simulink model "controller"  (R2022b)
settings: Solver=ode4  StartTime=0.0  StopTime=4  FixedStep=0.001  RelTol=1e-3
PreLoadFcn:
  | global m1 m2 l g m1_hat m2_hat;
  | m1 = 2;
  | m2 = 2;
  | m1_hat = 0.97*m1;
  | m2_hat = 0.97*m2;
  | l = 1;
  | g = 9.81;
  | 
  | kd = 200;
  | md = m1_hat;
  | dd = 2*0.7*sqrt(kd*md);
  | 
  | Kd = [kd,0;0,kd];
  | Md = [md,0;0,md];
  | Dd = [dd,0;0,dd];
  | 
  | p = 10^6;
  | d = 2*0.7*sqrt(p);
  | 
  | P = [p,0;0,p];
  | D = [d,0;0,d];
  | 
  | D_hold = D;
  | P_hold = P;
  | 
  | ke = 300;
  | Ke = [ke,0;0,0];
  | 
  | Fc = 1;
  | cv = 4;
  | 
  | delta = 0.01;
  | 
  | x0 = [0.95,0.95];
  | dx0 = [0;0];
  | 
  | n_pow = 0.001;
  | 
  | wall = 0.8;
  | 
  | delay = 2;
libraries: simulink x19, bbblueBasicLib x7
(part 1 of 2)
settings Model: SimulationMode=external  ExtModeTrigDuration=100  Creator=Nick  LastModifiedBy=ABL
settings SolverCC: PositivePriorityOrder=on  AutoInsertRateTranBlk=on  InsertRTBMode=Always
settings OptimizationCC: EnhancedBackFolding=on  PassReuseOutputArgsAs=Individual arguments  ZeroExternalMemoryAtStartup=off  ZeroInternalMemoryAtStartup=off  MaxStackSize=64  OptimizeBlockOrder=speed  DifferentSizesBufferReuse=on  OptimizationCustomize=off  EfficientTunableParamExpr=on
settings DebuggingCC: ParameterTunabilityLossMsg=error  UnconnectedInputMsg=warning  UnconnectedOutputMsg=warning  UnconnectedLineMsg=warning
settings HardwareCC: ProdBitPerPointer=32  ProdBitPerSizeT=32  ProdBitPerPtrDiffT=32  ProdLargestAtomicInteger=Long  ProdLargestAtomicFloat=Double  ProdWordSize=32  ProdHWDeviceType=ARM Compatible->ARM Cortex  UseEmbeddedCoderFeatures=off
settings ModelReferenceCC: EnableRefExpFcnMdlSchedulingChecks=on
settings SFSimCC: SimUserIncludeDirs=placeholders  MATLABDynamicMemAlloc=off
settings SFSimCC: SimCustomHeaderCode=|
  | #include "init_can.h"
  | #include "get_encoder.h"
  | #include "set_motor.h"
  | #include "print_input.h"
  | #include "stop_motor.h"
  | #include "datalog.h"
settings SFSimCC: SimUserSources=|
  | placeholders\init_can.c
  | placeholders\set_motor.c
  | placeholders\get_encoder.c
  | placeholders\print_input.c
  | placeholders\stop_motor.c
  | placeholders\datalog.c
settings RTWCC: Description=Embedded Coder  SystemTargetFile=ert.tlc  HardwareBoard=BeagleBone Blue  TLCOptions="-aInlineSetEventsForThisBaseRateFcn=TLC_FALSE -aSuppressMultiTaskScheduler=TLC_FALSE  -aRateBasedStepFcn=0"  TemplateMakefile=ert_default_tmf  RTWUseSimCustomCode=on  CustomInclude=placeholders  Toolchain=GNU GCC BeagleBone Blue  BuildConfiguration=Faster Runs  DLArmComputeVersion=19.05
settings RTWCC: CustomHeaderCode=|
  | #include "init_can.h"
  | #include "get_encoder.h"
  | #include "set_motor.h"
  | #include "print_input.h"
  | #include "stop_motor.h"
  | #include "datalog.h"
settings RTWCC: CustomSource=|
  | placeholders\init_can.c
  | placeholders\set_motor.c
  | placeholders\get_encoder.c
  | placeholders\print_input.c
  | placeholders\stop_motor.c
  | placeholders\datalog.c
settings CodeAppCC: ForceParamTrailComments=on  IgnoreCustomStorageClasses=off  OperatorAnnotations=on  SimulinkDataObjDesc=on  SFDataObjDesc=on  InsertBlockDesc=on
settings ERTTargetCC: SupportNonInlinedSFcns=on  SupportVariableSizeSignals=on

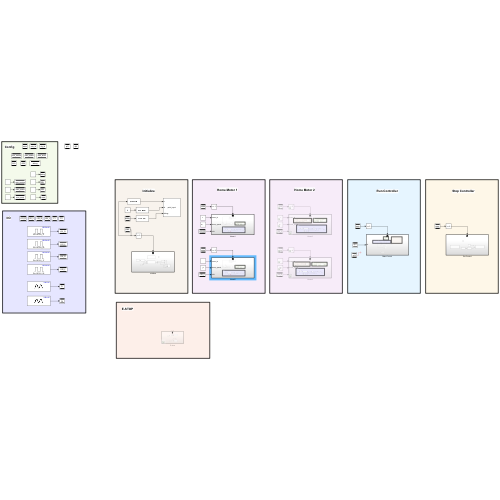
[thumbnail: Simulink's stored preview of the top-level diagram]
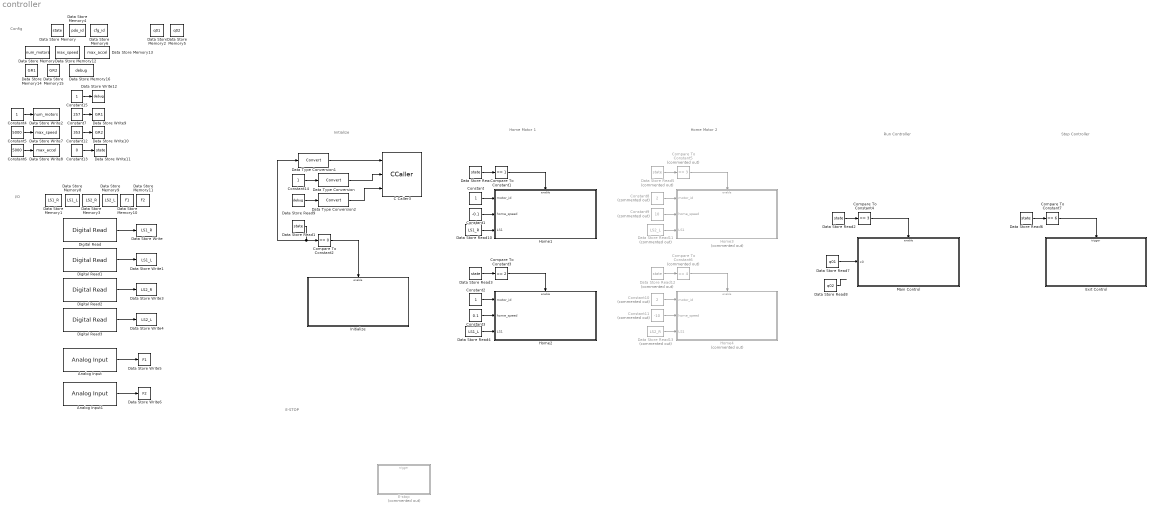
== system controller ==
  note: E-STOP
  note: Run Controller
  note: Home Motor 1
  note: Initialize
  note: Config
  note: I/O
  note: Stop Controller
  note: Home Motor 2
  Analog Input : bbblueBasicLib/Analog Input  Pin=AIN0  Mode=Raw  SampleTime=0.1  SimulateUsing=Code generation
  Analog Input1 : bbblueBasicLib/Analog Input  Pin=AIN0  Mode=Raw  SampleTime=0.1  SimulateUsing=Code generation
  C Caller3 : CCaller  FunctionName=print_input  PortSpecificationStruct="%)30     .    : 4   8    (     @         %    \"     ,    !     0         %  0 \"0    $    _    07)G3F%M90  4&]R=$YA;64 4V-O<&4     26YD97@     5'EP90      4VEZ90      27-';&]B86P   X    P    !@    @    $          4    (     0    $    !         !   0!A    #@   #     &    \"     0         !0    @    !     0    $         $  ! &$    .    .     8    (    !          %    \"     $    %     0         0    !0   $EN<'5T    #@   #@    &    \"     8         !0    @    !     0    $         \"0    @               X    X    !@    @    $          4    (     0    4    !         !     %    :6YT,S(    .    ,     8    (    !          %    \"     $    !     0         0  $ ,0    X    P    !@    @    ) @        4    (     0    $    !          (  0      #@   #     &    \"     0         !0    @    !     @    $         $  \" &ED   .    ,     8    (    !          %    \"     $    \"     0         0  ( :60   X    X    !@    @    $          4    (     0    4    !         !     %    26YP=70    .    .     8    (    !@         %    \"     $    !     0         )    \"            / _#@   #@    &    \"     0         !0    @    !    !0    $         $     4   !I;G0S,@    X    P    !@    @    $          4    (     0    $    !         !   0 Q    #@   #     &    \"     D\"        !0    @    !     0    $          @ !       .    .     8    (    !          %    \"     $    %     0         0    !0   &1E8G5G    #@   #@    &    \"     0         !0    @    !    !0    $         $     4   !D96)U9P    X    X    !@    @    $          4    (     0    4    !         !     %    26YP=70    .    .     8    (    !@         %    \"     $    !     0         )    \"             ! #@   #@    &    \"     0         !0    @    !    !0    $         $     4   !I;G0S,@    X    P    !@    @    $          4    (     0    $    !         !   0 Q    #@   #     &    \"     D\"        !0    @    !     0    $          @ !"  SampleTime=1
  Compare To Constant1 : simulink/Logic and Bit Operations/Compare To Constant  relop===  const=1  OutDataTypeStr=boolean
  Compare To Constant2 : simulink/Logic and Bit Operations/Compare To Constant  relop===  const=0  OutDataTypeStr=boolean
  Compare To Constant3 : simulink/Logic and Bit Operations/Compare To Constant  relop===  const=2  OutDataTypeStr=boolean
  Compare To Constant4 : simulink/Logic and Bit Operations/Compare To Constant  relop===  const=3  OutDataTypeStr=boolean
  Compare To Constant5 : simulink/Logic and Bit Operations/Compare To Constant  Commented=on  relop===  const=3  OutDataTypeStr=boolean
  Compare To Constant6 : simulink/Logic and Bit Operations/Compare To Constant  Commented=on  relop===  const=4  OutDataTypeStr=boolean
  Compare To Constant7 : simulink/Logic and Bit Operations/Compare To Constant  relop===  const=6  OutDataTypeStr=boolean
  Constant{,2,4,14..15} (5 alike) : Constant
  Constant1 : Constant  Value=-0.1
  Constant10 : Constant  Commented=on  Value=2
  Constant11 : Constant  Commented=on  Value=-10
  Constant12 : Constant  Value=353
  Constant13 : Constant  Value=0
  Constant3 : Constant  Value=0.1
  Constant5 : Constant  Value=5000
  Constant6 : Constant  Value=5000
  Constant7 : Constant  Value=257
  Constant8 : Constant  Commented=on  Value=2
  Constant9 : Constant  Commented=on  Value=10
  Data Store Memory : DataStoreMemory  DataStoreName=state  WriteAfterWriteMsg=warning  ShowAdditionalParam=off  OutDataTypeStr=double
  Data Store Memory1 : DataStoreMemory  DataStoreName=LS1_R  WriteAfterWriteMsg=warning  ShowAdditionalParam=off
  Data Store Memory10 : DataStoreMemory  DataStoreName=F1  WriteAfterWriteMsg=warning  ShowAdditionalParam=off
  Data Store Memory11 : DataStoreMemory  DataStoreName=F2  WriteAfterWriteMsg=warning  ShowAdditionalParam=off
  Data Store Memory12 : DataStoreMemory  DataStoreName=max_speed  WriteAfterWriteMsg=warning  ShowAdditionalParam=off
  Data Store Memory13 : DataStoreMemory  DataStoreName=max_accel  WriteAfterWriteMsg=warning  ShowAdditionalParam=off
  Data Store Memory14 : DataStoreMemory  DataStoreName=GR1  WriteAfterWriteMsg=warning  ShowAdditionalParam=off
  Data Store Memory15 : DataStoreMemory  DataStoreName=GR2  WriteAfterWriteMsg=warning  ShowAdditionalParam=off
  Data Store Memory16 : DataStoreMemory  DataStoreName=debug  WriteAfterWriteMsg=warning  ShowAdditionalParam=off
  Data Store Memory2 : DataStoreMemory  DataStoreName=q01  WriteAfterWriteMsg=warning  ShowAdditionalParam=off
  Data Store Memory3 : DataStoreMemory  DataStoreName=LS2_R  WriteAfterWriteMsg=warning  ShowAdditionalParam=off
  Data Store Memory4 : DataStoreMemory  DataStoreName=pdo_id  WriteAfterWriteMsg=warning  ShowAdditionalParam=off
  Data Store Memory5 : DataStoreMemory  DataStoreName=q02  WriteAfterWriteMsg=warning  ShowAdditionalParam=off
  Data Store Memory6 : DataStoreMemory  DataStoreName=cfg_id  WriteAfterWriteMsg=warning  ShowAdditionalParam=off
  Data Store Memory7 : DataStoreMemory  DataStoreName=num_motors  WriteAfterWriteMsg=warning  ShowAdditionalParam=off
  Data Store Memory8 : DataStoreMemory  DataStoreName=LS1_L  WriteAfterWriteMsg=warning  ShowAdditionalParam=off
  Data Store Memory9 : DataStoreMemory  DataStoreName=LS2_L  WriteAfterWriteMsg=warning  ShowAdditionalParam=off
  Data Store Read{,1..3,6} (5 alike) : DataStoreRead  DataStoreName=state  IndexOptions=Index vector (dialog)  Indices=1  OutputSizes=1
  Data Store Read10 : DataStoreRead  DataStoreName=LS1_R  IndexOptions=Index vector (dialog)  Indices=1  OutputSizes=1
  Data Store Read11 : DataStoreRead  Commented=on  DataStoreName=LS2_L  IndexOptions=Index vector (dialog)  Indices=1  OutputSizes=1
  Data Store Read12 : DataStoreRead  Commented=on  DataStoreName=state  IndexOptions=Index vector (dialog)  Indices=1  OutputSizes=1
  Data Store Read13 : DataStoreRead  Commented=on  DataStoreName=LS2_R  IndexOptions=Index vector (dialog)  Indices=1  OutputSizes=1
  Data Store Read4 : DataStoreRead  DataStoreName=LS1_L  IndexOptions=Index vector (dialog)  Indices=1  OutputSizes=1
  Data Store Read5 : DataStoreRead  Commented=on  DataStoreName=state  IndexOptions=Index vector (dialog)  Indices=1  OutputSizes=1
  Data Store Read7 : DataStoreRead  DataStoreName=q01  IndexOptions=Index vector (dialog)  Indices=1  OutputSizes=1
  Data Store Read8 : DataStoreRead  DataStoreName=q02  IndexOptions=Index vector (dialog)  Indices=1  OutputSizes=1
  Data Store Read9 : DataStoreRead  DataStoreName=debug  IndexOptions=Index vector (dialog)  Indices=1  OutputSizes=1
  Data Store Write : DataStoreWrite  DataStoreName=LS1_R  IndexOptions=Index vector (dialog)  Indices=1  OutputSizes=1
  Data Store Write1 : DataStoreWrite  DataStoreName=LS1_L  IndexOptions=Index vector (dialog)  Indices=1  OutputSizes=1
  Data Store Write10 : DataStoreWrite  DataStoreName=GR2  IndexOptions=Index vector (dialog)  Indices=1  OutputSizes=1
  Data Store Write11 : DataStoreWrite  DataStoreName=state  SampleTime=10000  IndexOptions=Index vector (dialog)  Indices=1  OutputSizes=1
  Data Store Write12 : DataStoreWrite  DataStoreName=debug  IndexOptions=Index vector (dialog)  Indices=1  OutputSizes=1
  Data Store Write2 : DataStoreWrite  DataStoreName=num_motors  IndexOptions=Index vector (dialog)  Indices=1  OutputSizes=1
  Data Store Write3 : DataStoreWrite  DataStoreName=LS2_R  IndexOptions=Index vector (dialog)  Indices=1  OutputSizes=1
  Data Store Write4 : DataStoreWrite  DataStoreName=LS2_L  IndexOptions=Index vector (dialog)  Indices=1  OutputSizes=1
  Data Store Write5 : DataStoreWrite  DataStoreName=F1  IndexOptions=Index vector (dialog)  Indices=1  OutputSizes=1
  Data Store Write6 : DataStoreWrite  DataStoreName=F2  IndexOptions=Index vector (dialog)  Indices=1  OutputSizes=1
  Data Store Write7 : DataStoreWrite  DataStoreName=max_speed  IndexOptions=Index vector (dialog)  Indices=1  OutputSizes=1
  Data Store Write8 : DataStoreWrite  DataStoreName=max_accel  IndexOptions=Index vector (dialog)  Indices=1  OutputSizes=1
  Data Store Write9 : DataStoreWrite  DataStoreName=GR1  IndexOptions=Index vector (dialog)  Indices=1  OutputSizes=1
  Data Type Conversion : DataTypeConversion  SaturateOnIntegerOverflow=off  RndMeth=Floor
  Data Type Conversion1 : DataTypeConversion  SaturateOnIntegerOverflow=off  RndMeth=Floor
  Data Type Conversion2 : DataTypeConversion  SaturateOnIntegerOverflow=off  RndMeth=Floor
  Digital Read : bbblueBasicLib/Digital Read  Pin=49  Direction=input  GPIOSelect=GPIO3_17  SampleTime=0.1
  Digital Read1 : bbblueBasicLib/Digital Read  Pin=49  Direction=input  GPIOSelect=GPIO3_20  SampleTime=0.1
  Digital Read2 : bbblueBasicLib/Digital Read  Pin=49  Direction=input  GPIOSelect=GPIO1_17  SampleTime=0.1
  Digital Read3 : bbblueBasicLib/Digital Read  Pin=49  Direction=input  GPIOSelect=GPIO1_25  SampleTime=0.1
  E-stop : Subsystem  Commented=on  TreatAsAtomicUnit=on
  Exit Control : Subsystem
  Home1 : Subsystem
  Home2 : Subsystem
  Home3 : Subsystem  Commented=on
  Home4 : Subsystem  Commented=on
  Initialize : Subsystem
  Main Control : Subsystem
  wires:
  Data Store Read/1 -> Compare To Constant1/1
  Compare To Constant1/1 -> Home1/Enable
  Compare To Constant2/1 -> Initialize/Enable
  Constant/1 -> Home1/1(motor_id)
  Constant1/1 -> Home1/2(home_speed)
  Data Store Read6/1 -> Compare To Constant7/1
  Compare To Constant7/1 -> Exit Control/Trigger
  Constant4/1 -> Data Store Write2/1
  Digital Read2/1 -> Data Store Write3/1
  Digital Read3/1 -> Data Store Write4/1
  Analog Input/1 -> Data Store Write5/1
  Analog Input1/1 -> Data Store Write6/1
  Constant5/1 -> Data Store Write7/1
  Constant6/1 -> Data Store Write8/1
  Data Store Read2/1 -> Compare To Constant4/1
  Compare To Constant4/1 -> Main Control/Enable
  Digital Read/1 -> Data Store Write/1
  Constant7/1 -> Data Store Write9/1
  Constant12/1 -> Data Store Write10/1
  Data Type Conversion/1 -> C Caller3/2
  Constant13/1 -> Data Store Write11/1
  Data Type Conversion1/1 -> C Caller3/1
  Digital Read1/1 -> Data Store Write1/1
  Data Store Read7/1 -> Main Control/1(x0)
  Data Store Read8/1 -> ?
  Constant15/1 -> Data Store Write12/1
  Constant14/1 -> Data Type Conversion/1
  Data Store Read9/1 -> Data Type Conversion2/1
  Data Type Conversion2/1 -> C Caller3/3
  Data Store Read10/1 -> Home1/3(LS1)
  Constant9/1 -> Home3/2(home_speed)
  Compare To Constant6/1 -> Home4/Enable
  Data Store Read13/1 -> Home4/3(LS1)
  Constant11/1 -> Home4/2(home_speed)
  Data Store Read11/1 -> Home3/3(LS1)
  Constant8/1 -> Home3/1(motor_id)
  Data Store Read12/1 -> Compare To Constant6/1
  Constant10/1 -> Home4/1(motor_id)
  Compare To Constant5/1 -> Home3/Enable
  Data Store Read5/1 -> Compare To Constant5/1
  Data Store Read1/1 -> Compare To Constant2/1, Data Type Conversion1/1
  Data Store Read3/1 -> Compare To Constant3/1
  Constant3/1 -> Home2/2(home_speed)
  Constant2/1 -> Home2/1(motor_id)
  Data Store Read4/1 -> Home2/3(LS1)
  Compare To Constant3/1 -> Home2/Enable

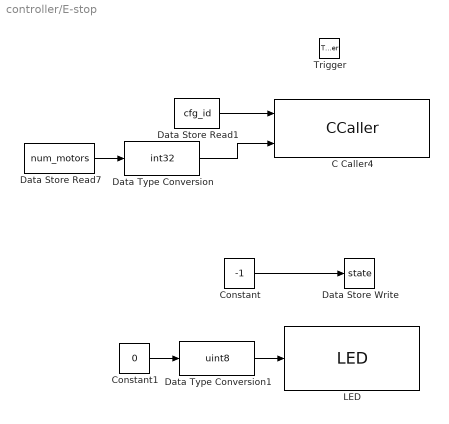
== system controller/E-stop ==
  Trigger : TriggerPort  VariantControl=(inherit)
  C Caller4 : CCaller  FunctionName=e_stop  PortSpecificationStruct="%)30     .    Z ,   8    (     @         %    \"     (    !     0         %  0 \"0    $    _    07)G3F%M90  4&]R=$YA;64 4V-O<&4     26YD97@     5'EP90      4VEZ90      27-';&]B86P   X    X    !@    @    $          4    (     0    8    !         !     &    8V9G7V9D   .    .     8    (    !          %    \"     $    &     0         0    !@   &-F9U]F9   #@   #@    &    \"     0         !0    @    !    !0    $         $     4   !);G!U=     X    X    !@    @    &          4    (     0    $    !          D    (               .    .     8    (    !          %    \"     $    %     0         0    !0   &EN=#,R    #@   #     &    \"     0         !0    @    !     0    $         $  ! #$    .    ,     8    (    \"0(        %    \"     $    !     0         \"  $       X   !     !@    @    $          4    (     0    H    !         !     *    ;G5M7VUO=&]R<P        X   !     !@    @    $          4    (     0    H    !         !     *    ;G5M7VUO=&]R<P        X    X    !@    @    $          4    (     0    4    !         !     %    26YP=70    .    .     8    (    !@         %    \"     $    !     0         )    \"            / _#@   #@    &    \"     0         !0    @    !    !0    $         $     4   !I;G0S,@    X    P    !@    @    $          4    (     0    $    !         !   0 Q    #@   #     &    \"     D\"        !0    @    !     0    $          @ !"
  Constant : Constant  Value=-1
  Constant1 : Constant  Value=0
  Data Store Read1 : DataStoreRead  DataStoreName=cfg_id  IndexOptions=Index vector (dialog)  Indices=1  OutputSizes=1
  Data Store Read7 : DataStoreRead  DataStoreName=num_motors  IndexOptions=Index vector (dialog)  Indices=1  OutputSizes=1
  Data Store Write : DataStoreWrite  DataStoreName=state  IndexOptions=Index vector (dialog)  Indices=1  OutputSizes=1
  Data Type Conversion : DataTypeConversion  OutDataTypeStr=int32  SaturateOnIntegerOverflow=off  RndMeth=Floor
  Data Type Conversion1 : DataTypeConversion  OutDataTypeStr=uint8  SaturateOnIntegerOverflow=off  RndMeth=Floor
  LED : bbblueBasicLib/LED  LED=Red
  wires:
  Data Store Read1/1 -> C Caller4/1
  Data Store Read7/1 -> Data Type Conversion/1
  Data Type Conversion/1 -> C Caller4/2
  Constant/1 -> Data Store Write/1
  Constant1/1 -> Data Type Conversion1/1
  Data Type Conversion1/1 -> LED/1

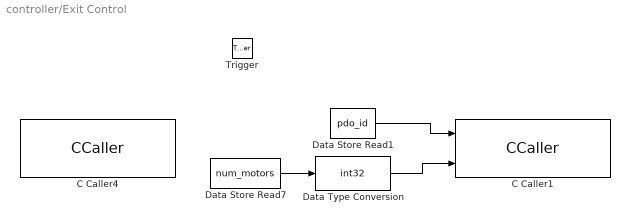
== system controller/Exit Control ==
  Trigger : TriggerPort  VariantControl=(inherit)  PortDimensions=1
  C Caller1 : CCaller  FunctionName=stop_motor  PortSpecificationStruct="%)30     .    Z ,   8    (     @         %    \"     (    !     0         %  0 \"0    $    _    07)G3F%M90  4&]R=$YA;64 4V-O<&4     26YD97@     5'EP90      4VEZ90      27-';&]B86P   X    X    !@    @    $          4    (     0    8    !         !     &    <&1O7V9D   .    .     8    (    !          %    \"     $    &     0         0    !@   '!D;U]F9   #@   #@    &    \"     0         !0    @    !    !0    $         $     4   !);G!U=     X    X    !@    @    &          4    (     0    $    !          D    (               .    .     8    (    !          %    \"     $    %     0         0    !0   &EN=#,R    #@   #     &    \"     0         !0    @    !     0    $         $  ! #$    .    ,     8    (    \"0(        %    \"     $    !     0         \"  $       X   !     !@    @    $          4    (     0    H    !         !     *    ;G5M7VUO=&]R<P        X   !     !@    @    $          4    (     0    H    !         !     *    ;G5M7VUO=&]R<P        X    X    !@    @    $          4    (     0    4    !         !     %    26YP=70    .    .     8    (    !@         %    \"     $    !     0         )    \"            / _#@   #@    &    \"     0         !0    @    !    !0    $         $     4   !I;G0S,@    X    P    !@    @    $          4    (     0    $    !         !   0 Q    #@   #     &    \"     D\"        !0    @    !     0    $          @ !"
  C Caller4 : CCaller  FunctionName=close_datalog
  Data Store Read1 : DataStoreRead  DataStoreName=pdo_id  IndexOptions=Index vector (dialog)  Indices=1  OutputSizes=1
  Data Store Read7 : DataStoreRead  DataStoreName=num_motors  IndexOptions=Index vector (dialog)  Indices=1  OutputSizes=1
  Data Type Conversion : DataTypeConversion  OutDataTypeStr=int32  SaturateOnIntegerOverflow=off  RndMeth=Floor
  wires:
  Data Type Conversion/1 -> C Caller1/2
  Data Store Read7/1 -> Data Type Conversion/1
  Data Store Read1/1 -> C Caller1/1

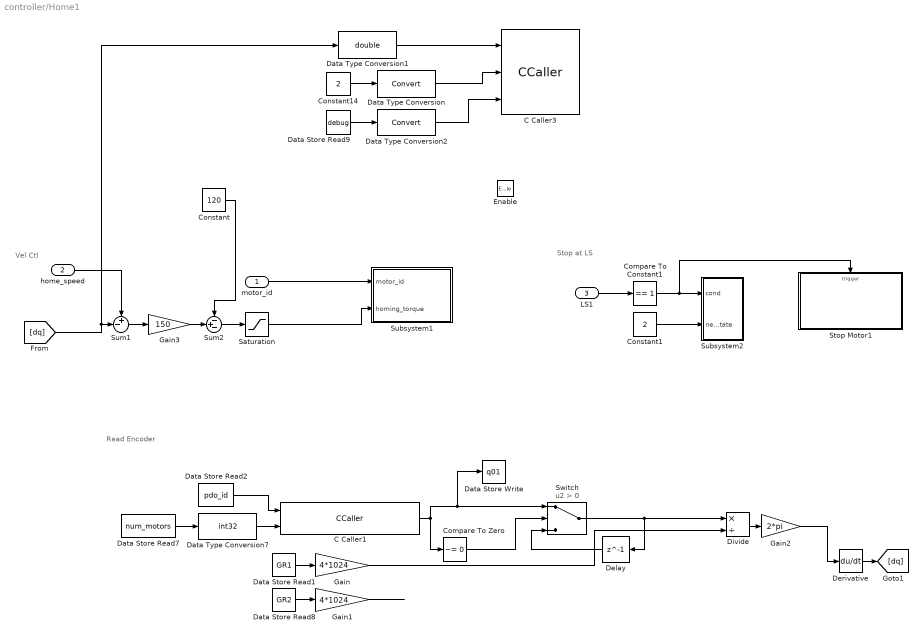
== system controller/Home1 ==
  note: Vel Ctl
  note: Read Encoder
  note: Stop at LS
  motor_id : Inport
  home_speed : Inport  Port=2
  LS1 : Inport  Port=3
  Enable : EnablePort
  C Caller1 : CCaller  FunctionName=get_encoder  PortSpecificationStruct="%)30     .    : 4   8    (     @         %    \"     ,    !     0         %  0 \"0    $    _    07)G3F%M90  4&]R=$YA;64 4V-O<&4     26YD97@     5'EP90      4VEZ90      27-';&]B86P   X    X    !@    @    $          4    (     0    8    !         !     &    <&1O7VED   .    .     8    (    !          %    \"     $    &     0         0    !@   '!D;U]I9   #@   #@    &    \"     0         !0    @    !    !0    $         $     4   !);G!U=     X    X    !@    @    &          4    (     0    $    !          D    (               .    .     8    (    !          %    \"     $    %     0         0    !0   &EN=#,R    #@   #     &    \"     0         !0    @    !     0    $         $  ! #$    .    ,     8    (    \"0(        %    \"     $    !     0         \"  $       X    P    !@    @    $          4    (     0    0    !         !  ! !S:7IE#@   #     &    \"     0         !0    @    !    !     $         $  $ '-I>F4.    .     8    (    !          %    \"     $    %     0         0    !0   $EN<'5T    #@   #@    &    \"     8         !0    @    !     0    $         \"0    @           #P/PX    X    !@    @    $          4    (     0    4    !         !     %    :6YT,S(    .    ,     8    (    !          %    \"     $    !     0         0  $ ,0    X    P    !@    @    ) @        4    (     0    $    !          (  0      #@   #     &    \"     0         !0    @    !     P    $         $  # '!O<P .    ,     8    (    !          %    \"     $    #     0         0  , <&]S  X    X    !@    @    $          4    (     0    8    !         !     &    3W5T<'5T   .    .     8    (    !@         %    \"     $    !     0         )    \"               #@   #@    &    \"     0         !0    @    !    !@    $         $     8   !D;W5B;&4   X    P    !@    @    $          4    (     0    $    !         !   0 Q    #@   #     &    \"     D\"        !0    @    !     0    $          @ !"  SampleTime=0.001
  C Caller3 : CCaller  FunctionName=print_input  PortSpecificationStruct="%)30     .    : 4   8    (     @         %    \"     ,    !     0         %  0 \"0    $    _    07)G3F%M90  4&]R=$YA;64 4V-O<&4     26YD97@     5'EP90      4VEZ90      27-';&]B86P   X    P    !@    @    $          4    (     0    $    !         !   0!A    #@   #     &    \"     0         !0    @    !     0    $         $  ! &$    .    .     8    (    !          %    \"     $    %     0         0    !0   $EN<'5T    #@   #@    &    \"     8         !0    @    !     0    $         \"0    @               X    X    !@    @    $          4    (     0    8    !         !     &    9&]U8FQE   .    ,     8    (    !          %    \"     $    !     0         0  $ ,0    X    P    !@    @    ) @        4    (     0    $    !          (  0      #@   #     &    \"     0         !0    @    !     @    $         $  \" &ED   .    ,     8    (    !          %    \"     $    \"     0         0  ( :60   X    X    !@    @    $          4    (     0    4    !         !     %    26YP=70    .    .     8    (    !@         %    \"     $    !     0         )    \"            / _#@   #@    &    \"     0         !0    @    !    !0    $         $     4   !I;G0S,@    X    P    !@    @    $          4    (     0    $    !         !   0 Q    #@   #     &    \"     D\"        !0    @    !     0    $          @ !       .    .     8    (    !          %    \"     $    %     0         0    !0   &1E8G5G    #@   #@    &    \"     0         !0    @    !    !0    $         $     4   !D96)U9P    X    X    !@    @    $          4    (     0    4    !         !     %    26YP=70    .    .     8    (    !@         %    \"     $    !     0         )    \"             ! #@   #@    &    \"     0         !0    @    !    !0    $         $     4   !I;G0S,@    X    P    !@    @    $          4    (     0    $    !         !   0 Q    #@   #     &    \"     D\"        !0    @    !     0    $          @ !"  SampleTime=0.001
  Compare To Constant1 : simulink/Logic and Bit Operations/Compare To Constant  relop===  const=1  OutDataTypeStr=boolean
  Compare To Zero : simulink/Logic and Bit Operations/Compare To Zero  relop=~=  OutDataTypeStr=boolean
  Constant : Constant  Value=120
  Constant1 : Constant  Value=2
  Constant14 : Constant  Value=2
  Data Store Read1 : DataStoreRead  DataStoreName=GR1  IndexOptions=Index vector (dialog)  Indices=1  OutputSizes=1
  Data Store Read2 : DataStoreRead  DataStoreName=pdo_id  IndexOptions=Index vector (dialog)  Indices=1  OutputSizes=1
  Data Store Read7 : DataStoreRead  DataStoreName=num_motors  IndexOptions=Index vector (dialog)  Indices=1  OutputSizes=1
  Data Store Read8 : DataStoreRead  DataStoreName=GR2  IndexOptions=Index vector (dialog)  Indices=1  OutputSizes=1
  Data Store Read9 : DataStoreRead  DataStoreName=debug  IndexOptions=Index vector (dialog)  Indices=1  OutputSizes=1
  Data Store Write : DataStoreWrite  DataStoreName=q01  IndexOptions=Index vector (dialog)  Indices=1  OutputSizes=1
  Data Type Conversion : DataTypeConversion  SaturateOnIntegerOverflow=off  RndMeth=Floor
  Data Type Conversion1 : DataTypeConversion  OutDataTypeStr=double  SaturateOnIntegerOverflow=off  RndMeth=Floor
  Data Type Conversion2 : DataTypeConversion  SaturateOnIntegerOverflow=off  RndMeth=Floor
  Data Type Conversion7 : DataTypeConversion  OutDataTypeStr=int32  SaturateOnIntegerOverflow=off  RndMeth=Floor
  Delay : Delay  DelayLength=1  InitialCondition=0
  Derivative : Derivative
  Divide : Product  Inputs=*/
  Gain : Gain  Gain=4*1024
  Gain1 : Gain  Gain=4*1024
  Gain2 : Gain  Gain=2*pi
  Gain3 : Gain  Gain=150
  Saturation : Saturate  UpperLimit=350  LowerLimit=-350
  Stop Motor1 : Subsystem  TreatAsAtomicUnit=on
  Subsystem1 : Subsystem
  Subsystem2 : Subsystem
  Sum1 : Sum  Inputs=+-|
  Sum2 : Sum  Inputs=-+-
  Switch : Switch  Criteria=u2 > Threshold  SaturateOnIntegerOverflow=off  InputSameDT=off
  wires:
  motor_id/1 -> Subsystem1/1(motor_id)
  Data Store Read1/1 -> Gain/1
  Divide/1 -> Gain2/1
  Compare To Zero/1 -> Switch/2
  Data Store Read8/1 -> Gain1/1
  Delay/1 -> Switch/3
  Gain/1 -> Divide/2
  Gain1/1 -> ?
  Data Store Read2/1 -> C Caller1/1
  Switch/1 -> Delay/1, Divide/1
  Data Store Read7/1 -> Data Type Conversion7/1
  Data Type Conversion7/1 -> C Caller1/2
  home_speed/1 -> Sum1/1
  LS1/1 -> Compare To Constant1/1
  Constant1/1 -> Subsystem2/2(new_state)
  Compare To Constant1/1 -> Stop Motor1/Trigger, Subsystem2/1(cond)
  Data Type Conversion2/1 -> C Caller3/3
  Data Store Read9/1 -> Data Type Conversion2/1
  Constant14/1 -> Data Type Conversion/1
  Data Type Conversion/1 -> C Caller3/2
  Data Type Conversion1/1 -> C Caller3/1
  Derivative/1 -> [dq]
  Saturation/1 -> Subsystem1/2(homing_torque)
  Sum2/1 -> Saturation/1
  [dq] -> Data Type Conversion1/1, Sum1/2
  Sum1/1 -> Gain3/1
  Gain3/1 -> Sum2/2
  Constant/1 -> Sum2/1
  Gain2/1 -> Derivative/1
  C Caller1/1 -> Data Store Write/1, Switch/1, Compare To Zero/1

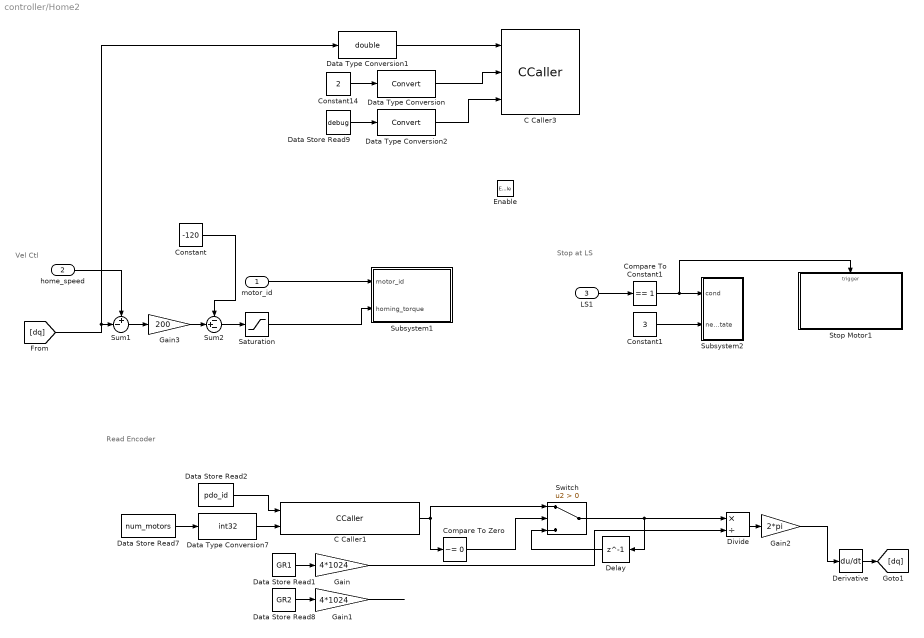
== system controller/Home2 ==
  note: Vel Ctl
  note: Read Encoder
  note: Stop at LS
  motor_id : Inport
  home_speed : Inport  Port=2
  LS1 : Inport  Port=3
  Enable : EnablePort
  C Caller1 : CCaller  FunctionName=get_encoder  PortSpecificationStruct="%)30     .    : 4   8    (     @         %    \"     ,    !     0         %  0 \"0    $    _    07)G3F%M90  4&]R=$YA;64 4V-O<&4     26YD97@     5'EP90      4VEZ90      27-';&]B86P   X    X    !@    @    $          4    (     0    8    !         !     &    <&1O7VED   .    .     8    (    !          %    \"     $    &     0         0    !@   '!D;U]I9   #@   #@    &    \"     0         !0    @    !    !0    $         $     4   !);G!U=     X    X    !@    @    &          4    (     0    $    !          D    (               .    .     8    (    !          %    \"     $    %     0         0    !0   &EN=#,R    #@   #     &    \"     0         !0    @    !     0    $         $  ! #$    .    ,     8    (    \"0(        %    \"     $    !     0         \"  $       X    P    !@    @    $          4    (     0    0    !         !  ! !S:7IE#@   #     &    \"     0         !0    @    !    !     $         $  $ '-I>F4.    .     8    (    !          %    \"     $    %     0         0    !0   $EN<'5T    #@   #@    &    \"     8         !0    @    !     0    $         \"0    @           #P/PX    X    !@    @    $          4    (     0    4    !         !     %    :6YT,S(    .    ,     8    (    !          %    \"     $    !     0         0  $ ,0    X    P    !@    @    ) @        4    (     0    $    !          (  0      #@   #     &    \"     0         !0    @    !     P    $         $  # '!O<P .    ,     8    (    !          %    \"     $    #     0         0  , <&]S  X    X    !@    @    $          4    (     0    8    !         !     &    3W5T<'5T   .    .     8    (    !@         %    \"     $    !     0         )    \"               #@   #@    &    \"     0         !0    @    !    !@    $         $     8   !D;W5B;&4   X    P    !@    @    $          4    (     0    $    !         !   0 Q    #@   #     &    \"     D\"        !0    @    !     0    $          @ !"  SampleTime=0.001
  C Caller3 : CCaller  FunctionName=print_input  PortSpecificationStruct="%)30     .    : 4   8    (     @         %    \"     ,    !     0         %  0 \"0    $    _    07)G3F%M90  4&]R=$YA;64 4V-O<&4     26YD97@     5'EP90      4VEZ90      27-';&]B86P   X    P    !@    @    $          4    (     0    $    !         !   0!A    #@   #     &    \"     0         !0    @    !     0    $         $  ! &$    .    .     8    (    !          %    \"     $    %     0         0    !0   $EN<'5T    #@   #@    &    \"     8         !0    @    !     0    $         \"0    @               X    X    !@    @    $          4    (     0    8    !         !     &    9&]U8FQE   .    ,     8    (    !          %    \"     $    !     0         0  $ ,0    X    P    !@    @    ) @        4    (     0    $    !          (  0      #@   #     &    \"     0         !0    @    !     @    $         $  \" &ED   .    ,     8    (    !          %    \"     $    \"     0         0  ( :60   X    X    !@    @    $          4    (     0    4    !         !     %    26YP=70    .    .     8    (    !@         %    \"     $    !     0         )    \"            / _#@   #@    &    \"     0         !0    @    !    !0    $         $     4   !I;G0S,@    X    P    !@    @    $          4    (     0    $    !         !   0 Q    #@   #     &    \"     D\"        !0    @    !     0    $          @ !       .    .     8    (    !          %    \"     $    %     0         0    !0   &1E8G5G    #@   #@    &    \"     0         !0    @    !    !0    $         $     4   !D96)U9P    X    X    !@    @    $          4    (     0    4    !         !     %    26YP=70    .    .     8    (    !@         %    \"     $    !     0         )    \"             ! #@   #@    &    \"     0         !0    @    !    !0    $         $     4   !I;G0S,@    X    P    !@    @    $          4    (     0    $    !         !   0 Q    #@   #     &    \"     D\"        !0    @    !     0    $          @ !"  SampleTime=0.001
  Compare To Constant1 : simulink/Logic and Bit Operations/Compare To Constant  relop===  const=1  OutDataTypeStr=boolean
  Compare To Zero : simulink/Logic and Bit Operations/Compare To Zero  relop=~=  OutDataTypeStr=boolean
  Constant : Constant  Value=-120
  Constant1 : Constant  Value=3
  Constant14 : Constant  Value=2
  Data Store Read1 : DataStoreRead  DataStoreName=GR1  IndexOptions=Index vector (dialog)  Indices=1  OutputSizes=1
  Data Store Read2 : DataStoreRead  DataStoreName=pdo_id  IndexOptions=Index vector (dialog)  Indices=1  OutputSizes=1
  Data Store Read7 : DataStoreRead  DataStoreName=num_motors  IndexOptions=Index vector (dialog)  Indices=1  OutputSizes=1
  Data Store Read8 : DataStoreRead  DataStoreName=GR2  IndexOptions=Index vector (dialog)  Indices=1  OutputSizes=1
  Data Store Read9 : DataStoreRead  DataStoreName=debug  IndexOptions=Index vector (dialog)  Indices=1  OutputSizes=1
  Data Type Conversion : DataTypeConversion  SaturateOnIntegerOverflow=off  RndMeth=Floor
  Data Type Conversion1 : DataTypeConversion  OutDataTypeStr=double  SaturateOnIntegerOverflow=off  RndMeth=Floor
  Data Type Conversion2 : DataTypeConversion  SaturateOnIntegerOverflow=off  RndMeth=Floor
  Data Type Conversion7 : DataTypeConversion  OutDataTypeStr=int32  SaturateOnIntegerOverflow=off  RndMeth=Floor
  Delay : Delay  DelayLength=1  InitialCondition=0
  Derivative : Derivative
  Divide : Product  Inputs=*/
  Gain : Gain  Gain=4*1024
  Gain1 : Gain  Gain=4*1024
  Gain2 : Gain  Gain=2*pi
  Gain3 : Gain  Gain=200
  Saturation : Saturate  UpperLimit=350  LowerLimit=-350
  Stop Motor1 : Subsystem  TreatAsAtomicUnit=on
  Subsystem1 : Subsystem
  Subsystem2 : Subsystem
  Sum1 : Sum  Inputs=+-|
  Sum2 : Sum  Inputs=-+-
  Switch : Switch  Criteria=u2 > Threshold  SaturateOnIntegerOverflow=off  InputSameDT=off
  wires:
  motor_id/1 -> Subsystem1/1(motor_id)
  Data Store Read1/1 -> Gain/1
  Divide/1 -> Gain2/1
  Compare To Zero/1 -> Switch/2
  Data Store Read8/1 -> Gain1/1
  Delay/1 -> Switch/3
  Gain/1 -> Divide/2
  Gain1/1 -> ?
  Gain2/1 -> Derivative/1
  C Caller1/1 -> Switch/1, Compare To Zero/1
  Data Store Read2/1 -> C Caller1/1
  Data Store Read7/1 -> Data Type Conversion7/1
  Data Type Conversion7/1 -> C Caller1/2
  home_speed/1 -> Sum1/1
  LS1/1 -> Compare To Constant1/1
  Constant1/1 -> Subsystem2/2(new_state)
  Compare To Constant1/1 -> Stop Motor1/Trigger, Subsystem2/1(cond)
  Data Type Conversion2/1 -> C Caller3/3
  Data Store Read9/1 -> Data Type Conversion2/1
  Constant14/1 -> Data Type Conversion/1
  Data Type Conversion/1 -> C Caller3/2
  Data Type Conversion1/1 -> C Caller3/1
  Derivative/1 -> [dq]
  Saturation/1 -> Subsystem1/2(homing_torque)
  Sum2/1 -> Saturation/1
  [dq] -> Data Type Conversion1/1, Sum1/2
  Sum1/1 -> Gain3/1
  Gain3/1 -> Sum2/2
  Constant/1 -> Sum2/1
  Switch/1 -> Delay/1, Divide/1

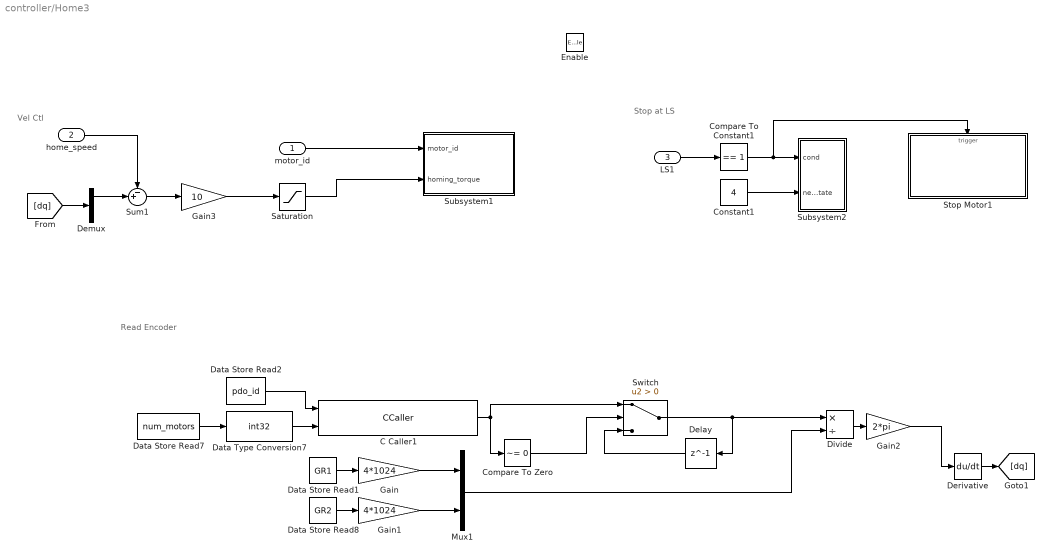
== system controller/Home3 ==
  note: Vel Ctl
  note: Read Encoder
  note: Stop at LS
  motor_id : Inport
  home_speed : Inport  Port=2
  LS1 : Inport  Port=3
  Enable : EnablePort
  C Caller1 : CCaller  FunctionName=get_encoder  PortSpecificationStruct="%)30     .    : 4   8    (     @         %    \"     ,    !     0         %  0 \"0    $    _    07)G3F%M90  4&]R=$YA;64 4V-O<&4     26YD97@     5'EP90      4VEZ90      27-';&]B86P   X    X    !@    @    $          4    (     0    8    !         !     &    <&1O7VED   .    .     8    (    !          %    \"     $    &     0         0    !@   '!D;U]I9   #@   #@    &    \"     0         !0    @    !    !0    $         $     4   !);G!U=     X    X    !@    @    &          4    (     0    $    !          D    (               .    .     8    (    !          %    \"     $    %     0         0    !0   &EN=#,R    #@   #     &    \"     0         !0    @    !     0    $         $  ! #$    .    ,     8    (    \"0(        %    \"     $    !     0         \"  $       X    P    !@    @    $          4    (     0    0    !         !  ! !S:7IE#@   #     &    \"     0         !0    @    !    !     $         $  $ '-I>F4.    .     8    (    !          %    \"     $    %     0         0    !0   $EN<'5T    #@   #@    &    \"     8         !0    @    !     0    $         \"0    @           #P/PX    X    !@    @    $          4    (     0    4    !         !     %    :6YT,S(    .    ,     8    (    !          %    \"     $    !     0         0  $ ,0    X    P    !@    @    ) @        4    (     0    $    !          (  0      #@   #     &    \"     0         !0    @    !     P    $         $  # '!O<P .    ,     8    (    !          %    \"     $    #     0         0  , <&]S  X    X    !@    @    $          4    (     0    8    !         !     &    3W5T<'5T   .    .     8    (    !@         %    \"     $    !     0         )    \"               #@   #@    &    \"     0         !0    @    !    !@    $         $     8   !D;W5B;&4   X    P    !@    @    $          4    (     0    $    !         !   0 R    #@   #     &    \"     D\"        !0    @    !     0    $          @ !"  SampleTime=0.001
  Compare To Constant1 : simulink/Logic and Bit Operations/Compare To Constant  relop===  const=1  OutDataTypeStr=boolean
  Compare To Zero : simulink/Logic and Bit Operations/Compare To Zero  relop=~=  OutDataTypeStr=boolean
  Constant1 : Constant  Value=4
  Data Store Read1 : DataStoreRead  DataStoreName=GR1  IndexOptions=Index vector (dialog)  Indices=1  OutputSizes=1
  Data Store Read2 : DataStoreRead  DataStoreName=pdo_id  IndexOptions=Index vector (dialog)  Indices=1  OutputSizes=1
  Data Store Read7 : DataStoreRead  DataStoreName=num_motors  IndexOptions=Index vector (dialog)  Indices=1  OutputSizes=1
  Data Store Read8 : DataStoreRead  DataStoreName=GR2  IndexOptions=Index vector (dialog)  Indices=1  OutputSizes=1
  Data Type Conversion7 : DataTypeConversion  OutDataTypeStr=int32  SaturateOnIntegerOverflow=off  RndMeth=Floor
  Delay : Delay  DelayLength=1  InitialCondition=0
  Demux : Demux  Outputs=2
  Derivative : Derivative
  Divide : Product  Inputs=*/
  Gain : Gain  Gain=4*1024
  Gain1 : Gain  Gain=4*1024
  Gain2 : Gain  Gain=2*pi
  Gain3 : Gain  Gain=10
  Mux1 : Mux  Inputs=2
  Saturation : Saturate  UpperLimit=30  LowerLimit=-30
  Stop Motor1 : Subsystem  TreatAsAtomicUnit=on
  Subsystem1 : Subsystem
  Subsystem2 : Subsystem
  Sum1 : Sum  Inputs=-+|
  Switch : Switch  Criteria=u2 > Threshold  SaturateOnIntegerOverflow=off  InputSameDT=off
  wires:
  motor_id/1 -> Subsystem1/1(motor_id)
  Derivative/1 -> [dq]
  Data Store Read1/1 -> Gain/1
  Divide/1 -> Gain2/1
  Compare To Zero/1 -> Switch/2
  Data Store Read8/1 -> Gain1/1
  Delay/1 -> Switch/3
  Mux1/1 -> Divide/2
  Gain1/1 -> Mux1/2
  Gain/1 -> Mux1/1
  Gain2/1 -> Derivative/1
  C Caller1/1 -> Switch/1, Compare To Zero/1
  Data Store Read2/1 -> C Caller1/1
  Switch/1 -> Delay/1, Divide/1
  Data Store Read7/1 -> Data Type Conversion7/1
  Data Type Conversion7/1 -> C Caller1/2
  [dq] -> Demux/1
  home_speed/1 -> Sum1/1
  Sum1/1 -> Gain3/1
  Gain3/1 -> Saturation/1
  Saturation/1 -> Subsystem1/2(homing_torque)
  Demux/1 -> Sum1/2
  Compare To Constant1/1 -> Stop Motor1/Trigger, Subsystem2/1(cond)
  Constant1/1 -> Subsystem2/2(new_state)
  LS1/1 -> Compare To Constant1/1

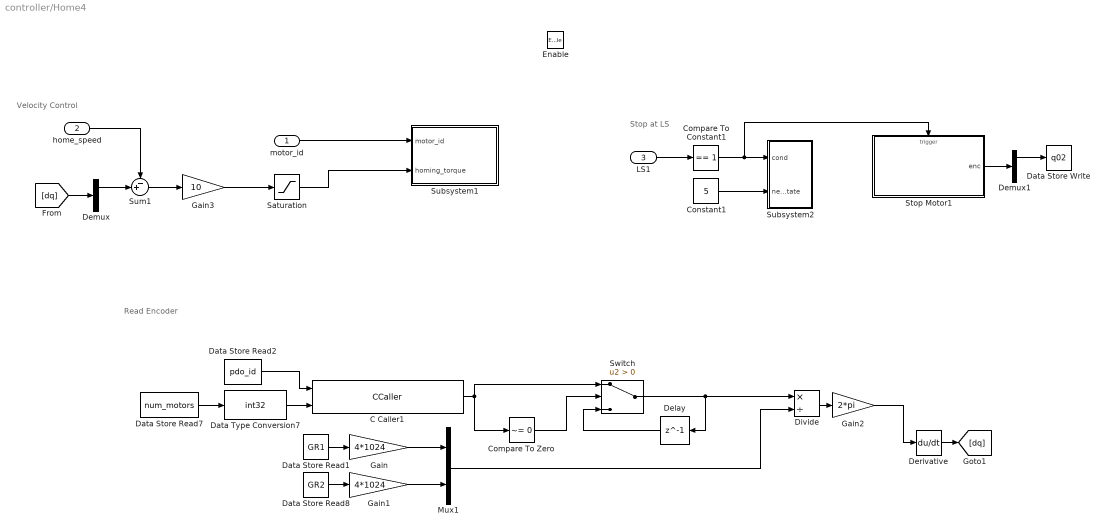
== system controller/Home4 ==
  note: Velocity Control
  note: Read Encoder
  note: Stop at LS
  motor_id : Inport
  home_speed : Inport  Port=2
  LS1 : Inport  Port=3
  Enable : EnablePort
  C Caller1 : CCaller  FunctionName=get_encoder  PortSpecificationStruct="%)30     .    : 4   8    (     @         %    \"     ,    !     0         %  0 \"0    $    _    07)G3F%M90  4&]R=$YA;64 4V-O<&4     26YD97@     5'EP90      4VEZ90      27-';&]B86P   X    X    !@    @    $          4    (     0    8    !         !     &    <&1O7VED   .    .     8    (    !          %    \"     $    &     0         0    !@   '!D;U]I9   #@   #@    &    \"     0         !0    @    !    !0    $         $     4   !);G!U=     X    X    !@    @    &          4    (     0    $    !          D    (               .    .     8    (    !          %    \"     $    %     0         0    !0   &EN=#,R    #@   #     &    \"     0         !0    @    !     0    $         $  ! #$    .    ,     8    (    \"0(        %    \"     $    !     0         \"  $       X    P    !@    @    $          4    (     0    0    !         !  ! !S:7IE#@   #     &    \"     0         !0    @    !    !     $         $  $ '-I>F4.    .     8    (    !          %    \"     $    %     0         0    !0   $EN<'5T    #@   #@    &    \"     8         !0    @    !     0    $         \"0    @           #P/PX    X    !@    @    $          4    (     0    4    !         !     %    :6YT,S(    .    ,     8    (    !          %    \"     $    !     0         0  $ ,0    X    P    !@    @    ) @        4    (     0    $    !          (  0      #@   #     &    \"     0         !0    @    !     P    $         $  # '!O<P .    ,     8    (    !          %    \"     $    #     0         0  , <&]S  X    X    !@    @    $          4    (     0    8    !         !     &    3W5T<'5T   .    .     8    (    !@         %    \"     $    !     0         )    \"               #@   #@    &    \"     0         !0    @    !    !@    $         $     8   !D;W5B;&4   X    P    !@    @    $          4    (     0    $    !         !   0 R    #@   #     &    \"     D\"        !0    @    !     0    $          @ !"  SampleTime=0.001
  Compare To Constant1 : simulink/Logic and Bit Operations/Compare To Constant  relop===  const=1  OutDataTypeStr=boolean
  Compare To Zero : simulink/Logic and Bit Operations/Compare To Zero  relop=~=  OutDataTypeStr=boolean
  Constant1 : Constant  Value=5
  Data Store Read1 : DataStoreRead  DataStoreName=GR1  IndexOptions=Index vector (dialog)  Indices=1  OutputSizes=1
  Data Store Read2 : DataStoreRead  DataStoreName=pdo_id  IndexOptions=Index vector (dialog)  Indices=1  OutputSizes=1
  Data Store Read7 : DataStoreRead  DataStoreName=num_motors  IndexOptions=Index vector (dialog)  Indices=1  OutputSizes=1
  Data Store Read8 : DataStoreRead  DataStoreName=GR2  IndexOptions=Index vector (dialog)  Indices=1  OutputSizes=1
  Data Store Write : DataStoreWrite  DataStoreName=q02  IndexOptions=Index vector (dialog)  Indices=1  OutputSizes=1
  Data Type Conversion7 : DataTypeConversion  OutDataTypeStr=int32  SaturateOnIntegerOverflow=off  RndMeth=Floor
  Delay : Delay  DelayLength=1  InitialCondition=0
  Demux : Demux  Outputs=2
  Demux1 : Demux  Outputs=2
  Derivative : Derivative
  Divide : Product  Inputs=*/
  Gain : Gain  Gain=4*1024
  Gain1 : Gain  Gain=4*1024
  Gain2 : Gain  Gain=2*pi
  Gain3 : Gain  Gain=10
  Mux1 : Mux  Inputs=2
  Saturation : Saturate  UpperLimit=30  LowerLimit=-30
  Stop Motor1 : Subsystem  TreatAsAtomicUnit=on
  Subsystem1 : Subsystem
  Subsystem2 : Subsystem
  Sum1 : Sum  Inputs=-+|
  Switch : Switch  Criteria=u2 > Threshold  SaturateOnIntegerOverflow=off  InputSameDT=off
  wires:
  motor_id/1 -> Subsystem1/1(motor_id)
  Derivative/1 -> [dq]
  Data Store Read1/1 -> Gain/1
  Divide/1 -> Gain2/1
  Compare To Zero/1 -> Switch/2
  Data Store Read8/1 -> Gain1/1
  Delay/1 -> Switch/3
  Mux1/1 -> Divide/2
  Gain1/1 -> Mux1/2
  Gain/1 -> Mux1/1
  Gain2/1 -> Derivative/1
  C Caller1/1 -> Switch/1, Compare To Zero/1
  Data Store Read2/1 -> C Caller1/1
  Switch/1 -> Delay/1, Divide/1
  Data Store Read7/1 -> Data Type Conversion7/1
  Data Type Conversion7/1 -> C Caller1/2
  [dq] -> Demux/1
  home_speed/1 -> Sum1/1
  Sum1/1 -> Gain3/1
  Gain3/1 -> Saturation/1
  Saturation/1 -> Subsystem1/2(homing_torque)
  Demux/1 -> Sum1/2
  Constant1/1 -> Subsystem2/2(new_state)
  Stop Motor1/1(enc) -> Demux1/1
  Demux1/1 -> Data Store Write/1
  Compare To Constant1/1 -> Stop Motor1/Trigger, Subsystem2/1(cond)
  LS1/1 -> Compare To Constant1/1

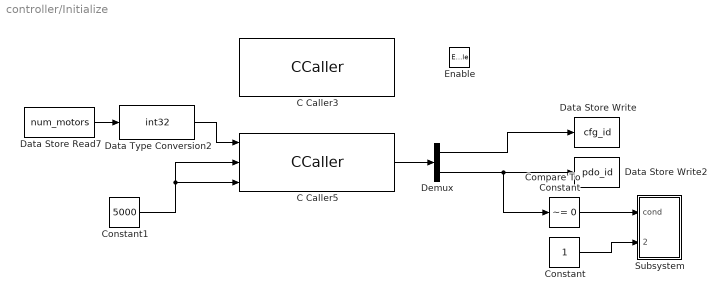
== system controller/Initialize ==
  Enable : EnablePort
  C Caller3 : CCaller  FunctionName=init_datalog  SampleTime=100
  C Caller5 : CCaller  FunctionName=init_can  PortSpecificationStruct="%)30     .    . <   8    (     @         %    \"     0    !     0         %  0 \"0    $    _    07)G3F%M90  4&]R=$YA;64 4V-O<&4     26YD97@     5'EP90      4VEZ90      27-';&]B86P   X   !     !@    @    $          4    (     0    H    !         !     *    ;G5M7VUO=&]R<P        X   !     !@    @    $          4    (     0    H    !         !     *    ;G5M7VUO=&]R<P        X    X    !@    @    $     ...(+2109 chars)"  SampleTime=10000
  Compare To Constant : simulink/Logic and Bit Operations/Compare To Constant  relop=~=  const=0  OutDataTypeStr=boolean
  Constant : Constant
  Constant1 : Constant  Value=5000
  Data Store Read7 : DataStoreRead  DataStoreName=num_motors  IndexOptions=Index vector (dialog)  Indices=1  OutputSizes=1
  Data Store Write : DataStoreWrite  DataStoreName=cfg_id  IndexOptions=Index vector (dialog)  Indices=1  OutputSizes=1
  Data Store Write2 : DataStoreWrite  DataStoreName=pdo_id  IndexOptions=Index vector (dialog)  Indices=1  OutputSizes=1
  Data Type Conversion2 : DataTypeConversion  OutDataTypeStr=int32  SaturateOnIntegerOverflow=off  RndMeth=Floor
  Demux : Demux  Outputs=2
  Subsystem : Subsystem
  wires:
  Compare To Constant/1 -> Subsystem/1(cond)
  Constant/1 -> Subsystem/2(new_state)
  Constant1/1 -> C Caller5/2, C Caller5/3
  C Caller5/1 -> Demux/1
  Demux/1 -> Data Store Write/1
  Demux/2 -> Compare To Constant/1, Data Store Write2/1
  Data Type Conversion2/1 -> C Caller5/1
  Data Store Read7/1 -> Data Type Conversion2/1
